simulink library "Meldas_library"  (R2018a)
settings: Solver=VariableStepAuto  StartTime=0.0  StopTime=10.0  RelTol=1e-3
values from neighbouring files (symbols this model uses):
  Cf = 19000    [Params.mat]
  Iz = 2875    [Params.mat]
  lf = 1.2    [Params.mat]
  m = 1575    [Params.mat]
settings Model: Creator=mulusoy  LastModifiedBy=mulusoy

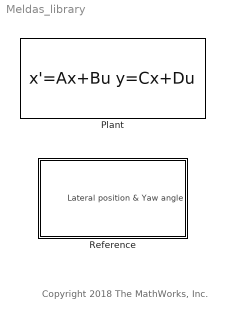
== system Meldas_library ==
  note: Copyright 2018 The MathWorks, Inc.
  Plant : StateSpace  A=|  B=[2*Cf/m 0 2*Cf*lf/Iz 0]';  C=[0 0 0 1; 0 1 0 0];  D=[0;0]  InitialCondition=0  mask{Vx=15}
      | [-(2*Cf+2*Cr)/m/Vx, 0, -Vx-(2*Cf*lf-2*Cr*lr)/m/Vx, 0;
      |      0, 0, 1, 0;
      |      -(2*Cf*lf-2*Cr*lr)/Iz/Vx, 0, -(2*Cf*lf^2+2*Cr*lr^2)/Iz/Vx, 0;
      |      1, Vx, 0, 0];
      mask Display: image("Car.jpg")
  Reference : Subsystem
      mask Display: image("Reference.jpg");

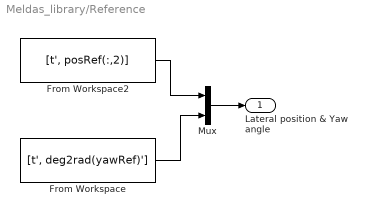
== system Meldas_library/Reference ==
  From Workspace : FromWorkspace  VariableName=[t', deg2rad(yawRef)']  SampleTime=0.1
  From Workspace2 : FromWorkspace  VariableName=[t', posRef(:,2)]  SampleTime=0.1
  Mux : Mux  Inputs=2
  Lateral position & Yaw angle : Outport
  wires:
  Mux/1 -> Lateral position & Yaw angle/1
  From Workspace/1 -> Mux/2
  From Workspace2/1 -> Mux/1
